simulink model "Copy_of_btp_pid"  (R2022a)
settings: Solver=ode4  StartTime=0.0  StopTime=0.2  FixedStep=0.001  RelTol=1e-3  EnableMultiTasking=on
undefined symbols (not defined in the file or in its folder): DiscIntNeverNeededParam
libraries: simulink x1, rllib x1
settings Model: Creator=sneha  LastModifiedBy=archi
settings SolverCC: AlgebraicLoopSolver=TrustRegion
settings DataIOCC: LimitDataPoints=on  SaveFormat=Array
settings OptimizationCC: LifeSpan=inf
settings DebuggingCC: UnconnectedInputMsg=warning  UnconnectedOutputMsg=warning  UnconnectedLineMsg=warning  SFUnexpectedBacktrackingDiag=warning  SFNoUnconditionalDefaultTransitionDiag=warning  SFExecutionAtInitializationDiag=none  SFMachineParentedDataDiag=warning  ArithmeticOperatorsInVariantConditions=warning
settings HardwareCC: ProdBitPerPointer=32  ProdBitPerSizeT=32  ProdBitPerPtrDiffT=32  ProdLargestAtomicFloat=None  ProdIntDivRoundTo=Undefined  ProdEndianess=Unspecified  ProdWordSize=32  ProdHWDeviceType=32-bit Generic
settings ModelReferenceCC: PropagateSignalLabelsOutOfModel=off
settings SFSimCC: SimUseLocalCustomCode=off  CustomCodeUndefinedFunction=UseInterfaceOnly
settings RTWCC: RTWUseLocalCustomCode=off
settings CodeAppCC: StateflowObjectComments=on
settings GRTTargetCC: TargetLangStandard=C89/C90 (ANSI)
settings ConfigComp: CovMetricSettings=dw  CovSaveCumulativeToWorkspaceVar=on  CovSaveSingleToWorkspaceVar=on  CovExternalEMLEnable=off

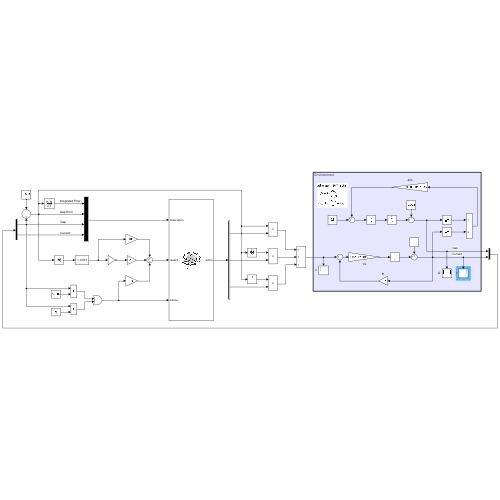
[thumbnail: Simulink's stored preview of the top-level diagram]
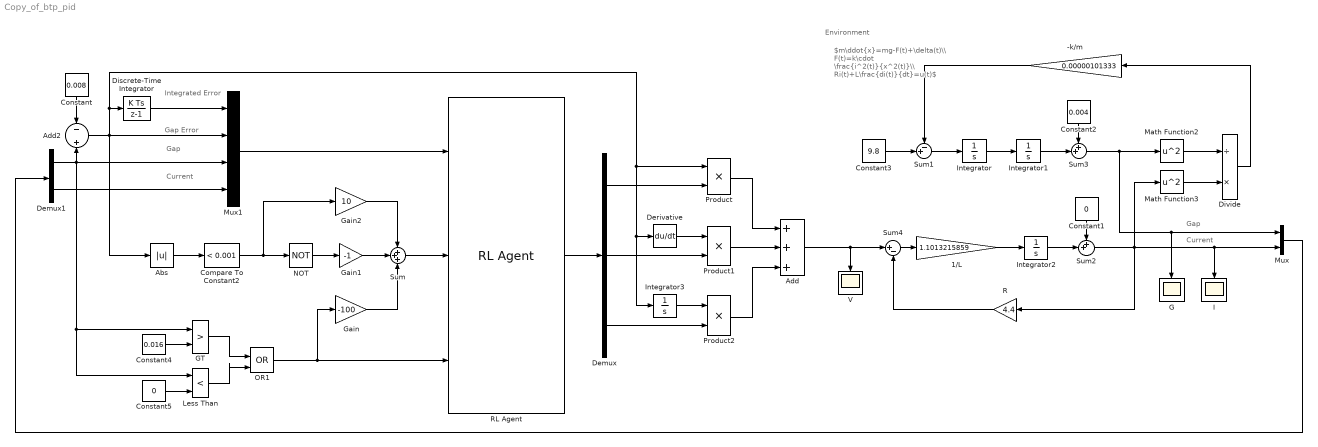
== system Copy_of_btp_pid ==
  note: $m\ddot{x}=mg-F(t)+\delta(t)\\ F(t)=k\cdot \frac{i^2(t)}{x^2(t)}\\ Ri(t)+L\frac{di(t)}{dt}=u(t)$
  note: Gap
  note: Environment
  note: Current
  note: Gap
  note: Gap Error
  note: Integrated Error
  note: Current
  -k/m : Gain  Gain=0.00000101333
  1/L : Gain  Gain=1.1013215859
  Abs : Abs  SaturateOnIntegerOverflow=off
  Add : Sum  Inputs=+++
  Add2 : Sum  Inputs=-|+
  Compare To Constant2 : simulink/Logic and Bit Operations/Compare To Constant  relop=<  const=0.001  OutDataTypeStr=boolean
  Constant : Constant  Value=0.008
  Constant1 : Constant  Value=0
  Constant2 : Constant  Value=0.004
  Constant3 : Constant  Value=9.8
  Constant4 : Constant  Value=0.016
  Constant5 : Constant  Value=0
  Demux : Demux  Outputs=3
  Demux1 : Demux  Outputs=2
  Derivative : Derivative
  Discrete-Time Integrator : DiscreteIntegrator  SampleTime=-1  ICPrevOutput=DiscIntNeverNeededParam  ICPrevScaledInput=DiscIntNeverNeededParam
  Divide : Product  Inputs=/*
  G : Scope
  GT : RelationalOperator  Operator=>  OutDataTypeStr=boolean  RndMeth=Simplest  InputSameDT=off
  Gain : Gain  Gain=-100
  Gain1 : Gain  Gain=-1
  Gain2 : Gain  Gain=10
  I : Scope
  Integrator{,1..3} (4 alike) : Integrator
  Less Than : RelationalOperator  Operator=<  OutDataTypeStr=boolean  RndMeth=Simplest  InputSameDT=off
  Math Function2 : Math  Operator=square
  Math Function3 : Math  Operator=square
  Mux : Mux  Inputs=2
  Mux1 : Mux
  NOT : Logic  Operator=NOT  IconShape=distinctive  AllPortsSameDT=off  OutDataTypeStr=boolean
  OR1 : Logic  Operator=OR  IconShape=distinctive  AllPortsSameDT=off  OutDataTypeStr=boolean
  Product : Product
  Product1 : Product
  Product2 : Product
  R : Gain  Gain=4.4
  RL Agent : rllib/RL Agent  Agent=rlDDPGAgent  ExternalActionAsInput=off  ProvideLastAction=off  ProvideCumRwd=off  TreatAsDirectFeedthrough=on  UseStrictObservationDataTypes=off
  Sum : Sum  Inputs=+++
  Sum1 : Sum  Inputs=-+|
  Sum2 : Sum  Inputs=++|
  Sum3 : Sum  Inputs=++|
  Sum4 : Sum  Inputs=|+-
  V : Scope
  wires:
  Math Function2/1 -> Divide/1
  Sum1/1 -> Integrator/1
  Math Function3/1 -> Divide/2
  -k/m/1 -> Sum1/1
  R/1 -> Sum4/2
  1/L/1 -> Integrator2/1
  Integrator/1 -> Integrator1/1
  Sum4/1 -> 1/L/1
  Divide/1 -> -k/m/1
  Constant3/1 -> Sum1/2
  Integrator2/1 -> Sum2/2
  Sum2/1 -> R/1, I/1, Mux/2, Math Function3/1
  Constant2/1 -> Sum3/1
  Integrator1/1 -> Sum3/2
  Constant1/1 -> Sum2/1
  Constant/1 -> Add2/1
  Mux1/1 -> RL Agent/1
  Constant4/1 -> GT/2
  Sum3/1 -> Math Function2/1, Mux/1, G/1
  Constant5/1 -> Less Than/2
  GT/1 -> OR1/1
  Less Than/1 -> OR1/2
  OR1/1 -> RL Agent/3, Gain/1
  Gain1/1 -> Sum/2
  Gain2/1 -> Sum/1
  NOT/1 -> Gain1/1
  Compare To Constant2/1 -> Gain2/1, NOT/1
  Gain/1 -> Sum/3
  Abs/1 -> Compare To Constant2/1
  Sum/1 -> RL Agent/2
  Discrete-Time Integrator/1 -> Mux1/1
  Demux/2 -> Product1/2
  Derivative/1 -> Product1/1
  Integrator3/1 -> Product2/1
  Product/1 -> Add/1
  Product2/1 -> Add/3
  Product1/1 -> Add/2
  Add2/1 -> Integrator3/1, Derivative/1, Product/1, Discrete-Time Integrator/1, Abs/1, Mux1/2
  RL Agent/1 -> Demux/1
  Demux/3 -> Product2/2
  Demux/1 -> Product/2
  Add/1 -> V/1, Sum4/1
  Mux/1 -> Demux1/1
  Demux1/2 -> Mux1/4
  Demux1/1 -> Less Than/1, GT/1, Add2/2, Mux1/3
